simulink model "HSimpleConst"  (Simulink 7.9)
settings: configuration reference "withOpts" (kept outside this file)
settings Model: Creator=boakes  LastModifiedBy=boakes
settings ConfigSet: SourceLocation=Base Workspace

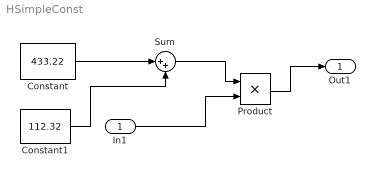
== system HSimpleConst ==
  In1 : Inport
  Constant : Constant  Value=433.22
  Constant1 : Constant  Value=112.32
  Product : Product  RndMeth=Zero
  Sum : Sum  Inputs=|++
  Out1 : Outport
  wires:
  Constant1/1 -> Sum/2
  In1/1 -> Product/2
  Product/1 -> Out1/1
  Constant/1 -> Sum/1
  Sum/1 -> Product/1
